simulink model "Simulation_model"  (R2022b)
settings: Solver=VariableStepAuto  StartTime=0.0  StopTime=12  RelTol=1e-3
values from neighbouring files (symbols this model uses):
  a1 = 1    [init_ff_vs_bs.m]
  a2 = 1    [init_ff_vs_bs.m]
  a3 = 1    [init_ff_vs_bs.m]
  b = 0.1    [init_ff_vs_bs.m]
  domega_max = 2*pi*n_max/60    (= 157.079632679)    [init_ff_vs_bs.m]
  dq0_d = dq0    [init_ff_vs_bs.m]
  Im = 740e-6    (= 0.00074)    [init_ff_vs_bs.m]
  Izz1 = (1/12)*m1*a1^2    (= 0.0833333333333)    [init_ff_vs_bs.m]
  Izz2 = (1/12)*m2*a2^2    (= 0.166666666667)    [init_ff_vs_bs.m]
  Izz3 = (1/12)*m3*a3^2    (= 0.25)    [init_ff_vs_bs.m]
  k_mot = 0.23    [init_ff_vs_bs.m]
  K_pid = 10    [init_ff_vs_bs.m]
  L = 50e-6    (= 5e-05)    [init_ff_vs_bs.m]
  q0 = [pi/2; -pi/3; 0]    [init_ff_vs_bs.m]
  q0_d = q0    [init_ff_vs_bs.m]
  R = 0.11    [init_ff_vs_bs.m]
  tau_max = 17.9    [init_ff_vs_bs.m]
  V_max = 48    [init_ff_vs_bs.m]
settings Model: Creator=rvitt  LastModifiedBy=rvitt

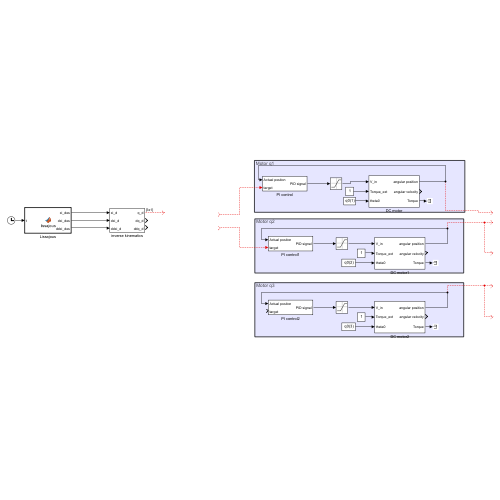
[thumbnail: Simulink's stored preview of the top-level diagram]
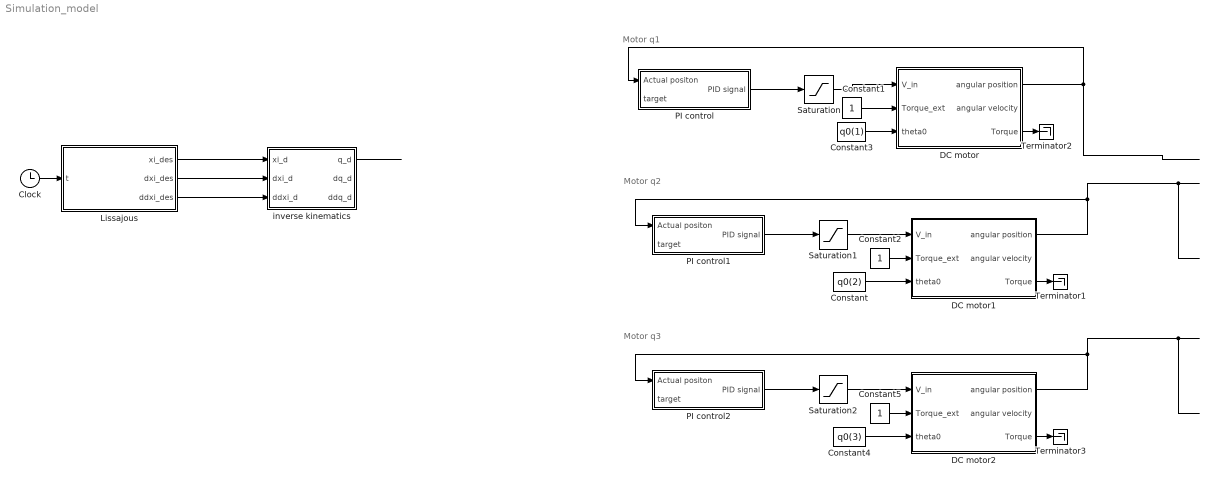
== system Simulation_model ==
  note: Motor q1
  note: Motor q2
  note: Motor q3
  Clock : Clock
  Constant : Constant  Value=q0(2)
  Constant1 : Constant
  Constant2 : Constant
  Constant3 : Constant  Value=q0(1)
  Constant4 : Constant  Value=q0(3)
  Constant5 : Constant
  DC motor : Subsystem
  DC motor1 : Subsystem
  DC motor2 : Subsystem
  Lissajous : MATLAB Function  TreatAsAtomicUnit=on
  PI control : Subsystem
  PI control1 : Subsystem
  PI control2 : Subsystem
  Saturation : Saturate  UpperLimit=V_max  LowerLimit=0
  Saturation1 : Saturate  UpperLimit=V_max  LowerLimit=0
  Saturation2 : Saturate  UpperLimit=V_max  LowerLimit=0
  Terminator1 : Terminator
  Terminator2 : Terminator
  Terminator3 : Terminator
  inverse kinematics : Subsystem
  wires:
  Constant1/1 -> DC motor/2(Torque_ext)
  PI control/1(PID signal) -> Saturation/1
  Saturation/1 -> DC motor/1(V_in)
  DC motor/1(angular position) -> PI control/1(Actual positon)
  DC motor/3(Torque) -> Terminator2/1
  DC motor1/1(angular position) -> PI control1/1(Actual positon)
  Saturation1/1 -> DC motor1/1(V_in)
  DC motor1/3(Torque) -> Terminator1/1
  PI control1/1(PID signal) -> Saturation1/1
  Constant2/1 -> DC motor1/2(Torque_ext)
  ? -> PI control/2(target)
  ? -> PI control1/2(target)
  Constant/1 -> DC motor1/3(theta0)
  Constant3/1 -> DC motor/3(theta0)
  Lissajous/1(xi_des) -> inverse kinematics/1(xi_d)
  Lissajous/2(dxi_des) -> inverse kinematics/2(dxi_d)
  Lissajous/3(ddxi_des) -> inverse kinematics/3(ddxi_d)
  Clock/1 -> Lissajous/1(t)
  inverse kinematics/1(q_d) -> ?
  Constant4/1 -> DC motor2/3(theta0)
  Constant5/1 -> DC motor2/2(Torque_ext)
  PI control2/1(PID signal) -> Saturation2/1
  DC motor2/3(Torque) -> Terminator3/1
  Saturation2/1 -> DC motor2/1(V_in)
  DC motor2/1(angular position) -> PI control2/1(Actual positon)

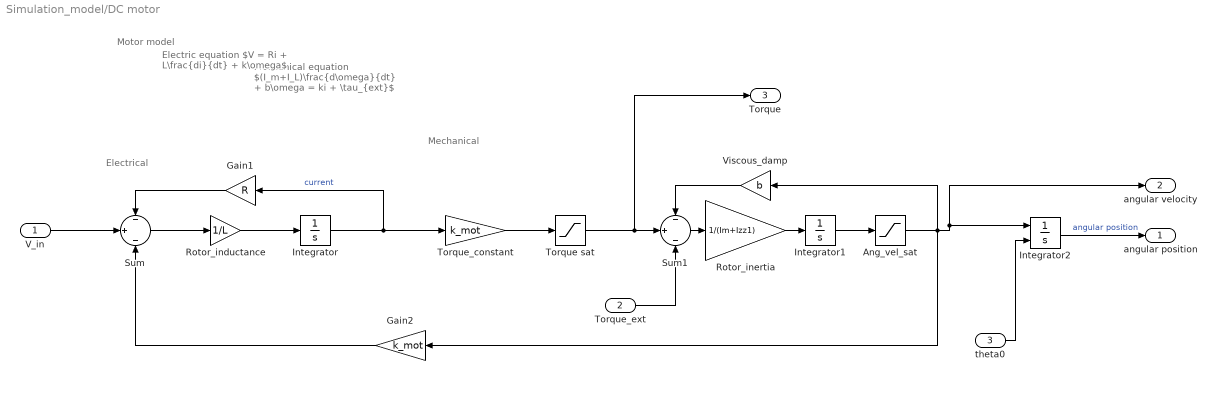
== system Simulation_model/DC motor ==
  note: Mechanical
  note: Electrical
  note: Motor model
  note: Mechanical equation
      | $(I_m+I_L)\frac{d\omega}{dt} + b\omega = ki + \tau_{ext}$
  note: Electric equation
      | $V = Ri + L\frac{di}{dt} + k\omega$
  V_in : Inport
  Torque_ext : Inport  Port=2
  theta0 : Inport  Port=3
  Ang_vel_sat : Saturate  UpperLimit=domega_max  LowerLimit=-domega_max
  Gain1 : Gain  Gain=R
  Gain2 : Gain  Gain=k_mot
  Integrator : Integrator
  Integrator1 : Integrator
  Integrator2 : Integrator  InitialConditionSource=external
  Rotor_inductance : Gain  Gain=1/L
  Rotor_inertia : Gain  Gain=1/(Im+Izz1)
  Sum : Sum  Inputs=-|+|-
  Sum1 : Sum  Inputs=-|+|-
  Torque sat : Saturate  UpperLimit=tau_max  LowerLimit=-tau_max
  Torque_constant : Gain  Gain=k_mot
  Viscous_damp : Gain  Gain=b
  angular position : Outport
  angular velocity : Outport  Port=2
  Torque : Outport  Port=3
  wires:
  Sum/1 -> Rotor_inductance/1
  Integrator/1 -> Gain1/1, Torque_constant/1  "current"
  Viscous_damp/1 -> Sum1/1
  Torque_ext/1 -> Sum1/3
  Sum1/1 -> Rotor_inertia/1
  Torque_constant/1 -> Torque sat/1
  Rotor_inductance/1 -> Integrator/1
  V_in/1 -> Sum/2
  Rotor_inertia/1 -> Integrator1/1
  Gain1/1 -> Sum/1
  Gain2/1 -> Sum/3
  Integrator2/1 -> angular position/1  "angular position"
  Integrator1/1 -> Ang_vel_sat/1
  Torque sat/1 -> Torque/1, Sum1/2
  Ang_vel_sat/1 -> Viscous_damp/1, angular velocity/1, Integrator2/1, Gain2/1
  theta0/1 -> Integrator2/2

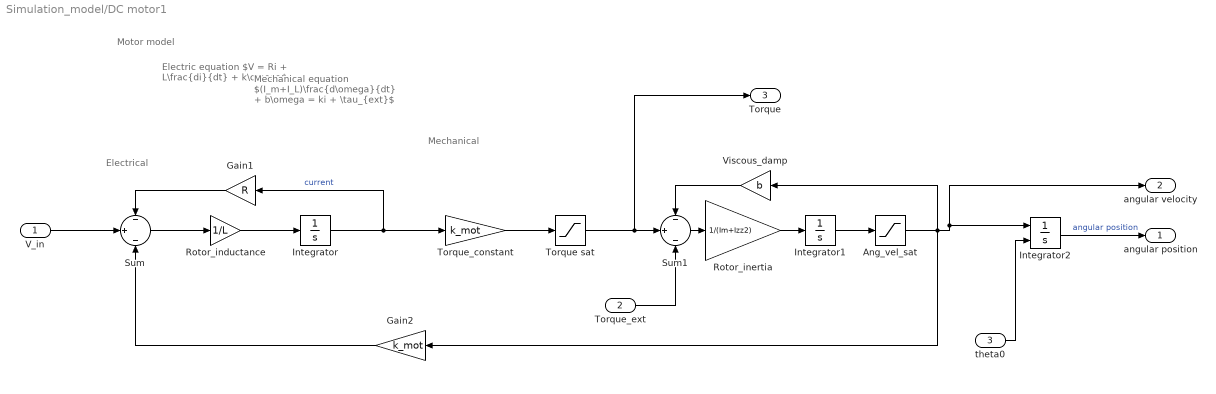
== system Simulation_model/DC motor1 ==
  note: Electric equation
      | $V = Ri + L\frac{di}{dt} + k\omega$
  note: Mechanical equation
      | $(I_m+I_L)\frac{d\omega}{dt} + b\omega = ki + \tau_{ext}$
  note: Motor model
  note: Electrical
  note: Mechanical
  V_in : Inport
  Torque_ext : Inport  Port=2
  theta0 : Inport  Port=3
  Ang_vel_sat : Saturate  UpperLimit=domega_max  LowerLimit=-domega_max
  Gain1 : Gain  Gain=R
  Gain2 : Gain  Gain=k_mot
  Integrator : Integrator
  Integrator1 : Integrator
  Integrator2 : Integrator  InitialConditionSource=external
  Rotor_inductance : Gain  Gain=1/L
  Rotor_inertia : Gain  Gain=1/(Im+Izz2)
  Sum : Sum  Inputs=-|+|-
  Sum1 : Sum  Inputs=-|+|-
  Torque sat : Saturate  UpperLimit=tau_max  LowerLimit=-tau_max
  Torque_constant : Gain  Gain=k_mot
  Viscous_damp : Gain  Gain=b
  angular position : Outport
  angular velocity : Outport  Port=2
  Torque : Outport  Port=3
  wires:
  theta0/1 -> Integrator2/2
  Ang_vel_sat/1 -> Gain2/1, Integrator2/1, angular velocity/1, Viscous_damp/1
  Torque sat/1 -> Sum1/2, Torque/1
  Integrator1/1 -> Ang_vel_sat/1
  Integrator2/1 -> angular position/1  "angular position"
  Gain2/1 -> Sum/3
  Gain1/1 -> Sum/1
  Rotor_inertia/1 -> Integrator1/1
  V_in/1 -> Sum/2
  Rotor_inductance/1 -> Integrator/1
  Torque_constant/1 -> Torque sat/1
  Sum1/1 -> Rotor_inertia/1
  Torque_ext/1 -> Sum1/3
  Viscous_damp/1 -> Sum1/1
  Integrator/1 -> Torque_constant/1, Gain1/1  "current"
  Sum/1 -> Rotor_inductance/1

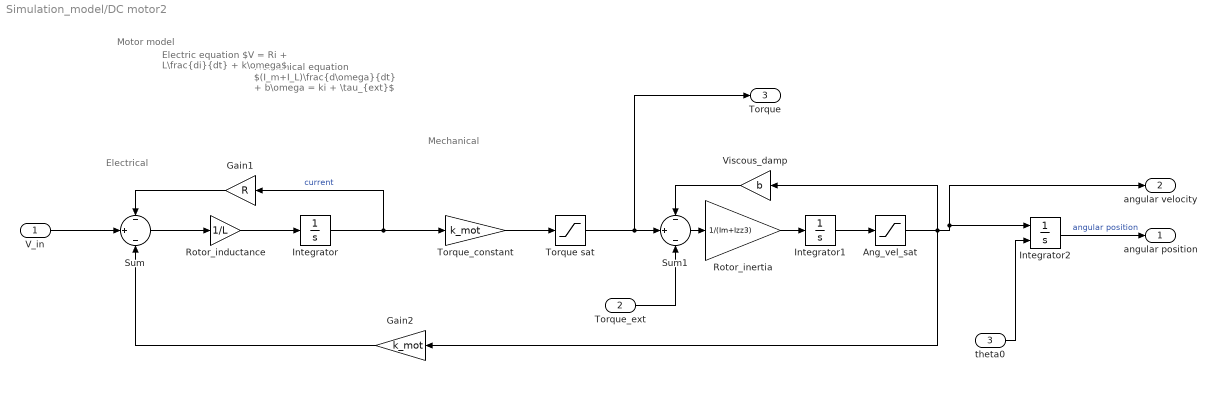
== system Simulation_model/DC motor2 ==
  note: Mechanical
  note: Electrical
  note: Motor model
  note: Mechanical equation
      | $(I_m+I_L)\frac{d\omega}{dt} + b\omega = ki + \tau_{ext}$
  note: Electric equation
      | $V = Ri + L\frac{di}{dt} + k\omega$
  V_in : Inport
  Torque_ext : Inport  Port=2
  theta0 : Inport  Port=3
  Ang_vel_sat : Saturate  UpperLimit=domega_max  LowerLimit=-domega_max
  Gain1 : Gain  Gain=R
  Gain2 : Gain  Gain=k_mot
  Integrator : Integrator
  Integrator1 : Integrator
  Integrator2 : Integrator  InitialConditionSource=external
  Rotor_inductance : Gain  Gain=1/L
  Rotor_inertia : Gain  Gain=1/(Im+Izz3)
  Sum : Sum  Inputs=-|+|-
  Sum1 : Sum  Inputs=-|+|-
  Torque sat : Saturate  UpperLimit=tau_max  LowerLimit=-tau_max
  Torque_constant : Gain  Gain=k_mot
  Viscous_damp : Gain  Gain=b
  angular position : Outport
  angular velocity : Outport  Port=2
  Torque : Outport  Port=3
  wires:
  Sum/1 -> Rotor_inductance/1
  Integrator/1 -> Gain1/1, Torque_constant/1  "current"
  Viscous_damp/1 -> Sum1/1
  Torque_ext/1 -> Sum1/3
  Sum1/1 -> Rotor_inertia/1
  Torque_constant/1 -> Torque sat/1
  Rotor_inductance/1 -> Integrator/1
  V_in/1 -> Sum/2
  Rotor_inertia/1 -> Integrator1/1
  Gain1/1 -> Sum/1
  Gain2/1 -> Sum/3
  Integrator2/1 -> angular position/1  "angular position"
  Integrator1/1 -> Ang_vel_sat/1
  Torque sat/1 -> Torque/1, Sum1/2
  Ang_vel_sat/1 -> Viscous_damp/1, angular velocity/1, Integrator2/1, Gain2/1
  theta0/1 -> Integrator2/2

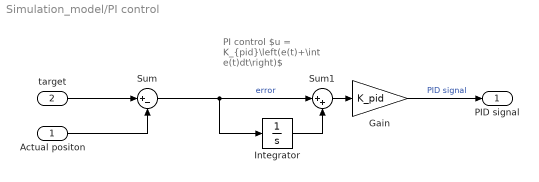
== system Simulation_model/PI control ==
  note: PI control
      | $u = K_{pid}\left(e(t)+\int e(t)dt\right)$
  Actual positon : Inport
  target : Inport  Port=2
  Gain : Gain  Gain=K_pid
  Integrator : Integrator
  Sum : Sum  Inputs=|+-
  Sum1 : Sum  Inputs=|++
  PID signal : Outport
  wires:
  Actual positon/1 -> Sum/2
  Sum1/1 -> Gain/1
  Gain/1 -> PID signal/1  "PID signal"
  Sum/1 -> Integrator/1, Sum1/1  "error"
  target/1 -> Sum/1
  Integrator/1 -> Sum1/2

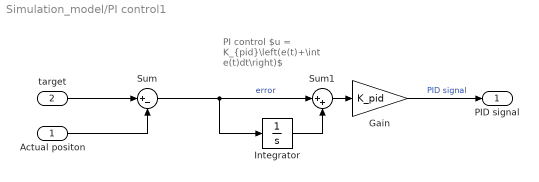
== system Simulation_model/PI control1 ==
  note: PI control
      | $u = K_{pid}\left(e(t)+\int e(t)dt\right)$
  Actual positon : Inport
  target : Inport  Port=2
  Gain : Gain  Gain=K_pid
  Integrator : Integrator
  Sum : Sum  Inputs=|+-
  Sum1 : Sum  Inputs=|++
  PID signal : Outport
  wires:
  Actual positon/1 -> Sum/2
  Sum1/1 -> Gain/1
  Gain/1 -> PID signal/1  "PID signal"
  Sum/1 -> Integrator/1, Sum1/1  "error"
  target/1 -> Sum/1
  Integrator/1 -> Sum1/2

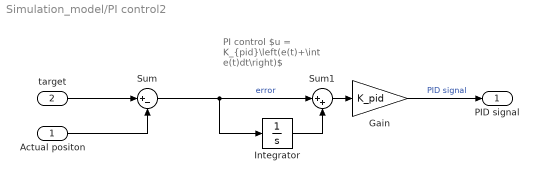
== system Simulation_model/PI control2 ==
  note: PI control
      | $u = K_{pid}\left(e(t)+\int e(t)dt\right)$
  Actual positon : Inport
  target : Inport  Port=2
  Gain : Gain  Gain=K_pid
  Integrator : Integrator
  Sum : Sum  Inputs=|+-
  Sum1 : Sum  Inputs=|++
  PID signal : Outport
  wires:
  Integrator/1 -> Sum1/2
  target/1 -> Sum/1
  Sum/1 -> Sum1/1, Integrator/1  "error"
  Gain/1 -> PID signal/1  "PID signal"
  Sum1/1 -> Gain/1
  Actual positon/1 -> Sum/2

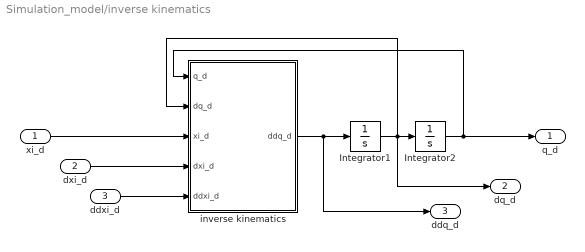
== system Simulation_model/inverse kinematics ==
  xi_d : Inport
  dxi_d : Inport  Port=2
  ddxi_d : Inport  Port=3
  Integrator1 : Integrator  InitialCondition=dq0_d
  Integrator2 : Integrator  InitialCondition=q0_d
  inverse kinematics : MATLAB Function  TreatAsAtomicUnit=on
  q_d : Outport  PortDimensions=[3,1]
  dq_d : Outport  Port=2  PortDimensions=[3,1]
  ddq_d : Outport  Port=3  PortDimensions=[3,1]
  wires:
  inverse kinematics/1(ddq_d) -> Integrator1/1, ddq_d/1
  Integrator2/1 -> inverse kinematics/1(q_d), q_d/1
  ddxi_d/1 -> inverse kinematics/5(ddxi_d)
  dxi_d/1 -> inverse kinematics/4(dxi_d)
  xi_d/1 -> inverse kinematics/3(xi_d)
  Integrator1/1 -> inverse kinematics/2(dq_d), Integrator2/1, dq_d/1

== matlab function Simulation_model/Lissajous ==
  data: t input; xi_des output size=[2,1]; dxi_des output size=[2,1]; ddxi_des output size=[2,1]; par_traj parameter
function [xi_des, dxi_des, ddxi_des] = lissajous(t, par_traj)

A = par_traj.A;
B = par_traj.B;
a = par_traj.a;
b = par_traj.b;
d = par_traj.d;
xi0 = par_traj.xi0;

xi_des = [A*sin(a*t+d); B*sin(b*t)] + xi0;
dxi_des = [A*a*cos(a*t+d); B*b*cos(b*t)];
ddxi_des = [-A*a^2*sin(a*t+d); -B*b^2*sin(b*t)];

== matlab function Simulation_model/inverse kinematics/inverse kinematics ==
  data: q_d input; dq_d input; xi_d input; dxi_d input; ddxi_d input; ddq_d output; a1 parameter; a3 parameter; a2 parameter
function ddq_d = fcn(q_d, dq_d, xi_d, dxi_d, ddxi_d, a1, a3, a2)

q1 = q_d(1);
q2 = q_d(2);
q3 = q_d(3);

dq1 = dq_d(1);
dq2 = dq_d(2);
dq3 = dq_d(3);

% Compute Jacobian
J =[-(a1*sin(q1+q2+q3)+a2*sin(q2+q3)+a3*sin(q3)), -(a2*sin(q2+q3)+a3*sin(q3)), -(a3*sin(q3));...
    a1*cos(q1+q2+q3)+a2*cos(q2+q3)+a3*cos(q3), a2*cos(q2+q3)+a3*cos(q3), a3*cos(q3)];

% jacobian derivative
J_dot = [-(a1*cos(q1+q2+q3)*(dq1+dq2+dq3)+a2*cos(q2+q3)*(dq2+dq3)+a3*sin(q3)*dq3), -(a2*cos(q2+q3)*(dq2+dq3)+a3*cos(q3)*dq3), -(a3*cos(q3)*dq3);
    -(a1*sin(q1+q2+q3)*(dq1+dq2+dq3)+a2*sin(q2+q3)*(dq2+dq3)+a3*sin(q3)*dq3), -(a2*sin(q2+q3)*(dq2+dq3)+a3*sin(q3)*dq3), -(a3*sin(q3)*dq3)];

% pseudoinverse
pinv_J = pinv(J,0.001);

% forward kinematics
p0 = [0; 0];
p1 = p0 + [a1*cos(q1); a1*sin(q1)];
p2 = p1 + [a2*cos(q1+q2); a2*sin(q1+q2)];
xi_curr = p2 + [a3*cos(q1+q2+q3); a3*cos(q1+q2+q3)];
dxi_curr = J*dq_d;

% second order CLIK
Kp = 100;
Kv = 30;
ddq_d = pinv_J * (ddxi_d - J_dot * dq_d + Kv*(dxi_d-dxi_curr) + Kp*(xi_d-xi_curr));
